simulink model "DQN_ABC_Test"  (R2023b)
settings: Solver=ode23tb  StartTime=0.0  StopTime=0.1  FixedStep=Ts  RelTol=1e-3
values from neighbouring files (symbols this model uses):
  Carm = 3.76    [DQn_ABC_Test_calc.m]
  L = Ld + Lm    [DQn_ABC_Test_calc.m]
  La = 1e-3    (= 0.001)    [DQn_ABC_Test_calc.m]
  Lb = 2*La    (= 0.002)    [DQn_ABC_Test_calc.m]
  Lc = 0.5*La    (= 0.0005)    [DQn_ABC_Test_calc.m]
  N = 1    [DQn_ABC_Test_calc.m]
  R = Rd + Rm    [DQn_ABC_Test_calc.m]
  Ra = 1.64    [DQn_ABC_Test_calc.m]
  Rb = 1.4*Ra    (= 2.296)    [DQn_ABC_Test_calc.m]
  Rc = 2.8*Ra    (= 4.592)    [DQn_ABC_Test_calc.m]
  Ta_dqn = oDP.Ta_dqn    [DQn_ABC_Test_calc.m]
  Ts = 50e-6    (= 5e-05)    [DQn_ABC_Test_calc.m]
  Ts_dqn = Ts    (= 5e-05)    [DQn_ABC_Test_calc.m]
  Ts_emt = Ts    (= 5e-05)    [DQn_ABC_Test_calc.m]
  Ws = 2*pi*f    (= 314.159265359)    [DQn_ABC_Test_calc.m]
undefined symbols (not defined in the file or in its folder): DiscIntNeverNeededParam, i, Xdcpnz, Xdcpnz_c, Xpnz, Ydcpnz, Ydcpnz_c, Ypnz
libraries: DQN_Lib x81, spsCurrentMeasurementLib x9, spsControlledVoltageSourceLib x9, spsSeriesRLCBranchLib x6, spsGroundLib x6, simulink x3, spsMutualInductanceLib x1, spspowerguiLib x1
(part 2 of 6)

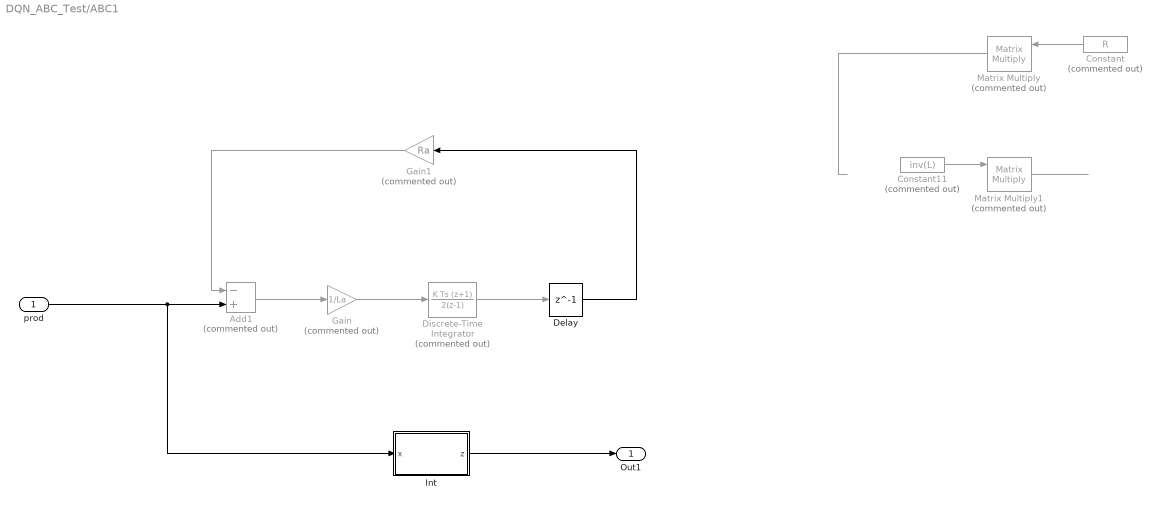
== system DQN_ABC_Test/ABC1 ==
  prod : Inport
  Add1 : Sum  Commented=on  Inputs=-+
  Constant : Constant  Commented=on  Value=R
  Constant11 : Constant  Commented=on  Value=inv(L)
  Delay : Delay  DelayLength=1
  Discrete-Time Integrator : DiscreteIntegrator  Commented=on  IntegratorMethod=Integration: Trapezoidal  SampleTime=Ts_emt  ICPrevOutput=DiscIntNeverNeededParam  ICPrevScaledInput=DiscIntNeverNeededParam
  Gain : Gain  Commented=on  Gain=1/La
  Gain1 : Gain  Commented=on  Gain=Ra
  Int : MATLAB Function  TreatAsAtomicUnit=on  mask{dt=Ts_emt}
      mask prompts: dt "Time step (s):"
  Matrix Multiply : Product  Commented=on  Multiplication=Matrix(*)
  Matrix Multiply1 : Product  Commented=on  Multiplication=Matrix(*)
  Out1 : Outport
  wires:
  prod/1 -> Int/1(x), Add1/2
  ? -> Matrix Multiply1/2
  Constant11/1 -> Matrix Multiply1/1
  Constant/1 -> Matrix Multiply/1
  Matrix Multiply1/1 -> ?
  Matrix Multiply/1 -> ?
  ? -> Matrix Multiply/2
  Add1/1 -> Gain/1
  Int/1(z) -> Out1/1
  Gain1/1 -> Add1/1
  Gain/1 -> Discrete-Time Integrator/1
  Discrete-Time Integrator/1 -> Delay/1
  Delay/1 -> Gain1/1

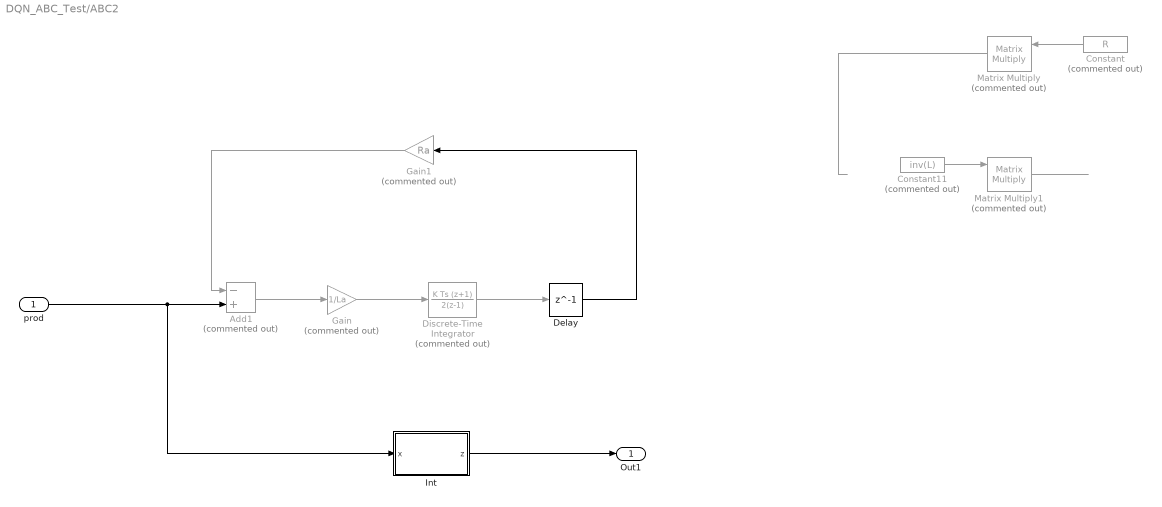
== system DQN_ABC_Test/ABC2 ==
  prod : Inport
  Add1 : Sum  Commented=on  Inputs=-+
  Constant : Constant  Commented=on  Value=R
  Constant11 : Constant  Commented=on  Value=inv(L)
  Delay : Delay  DelayLength=1
  Discrete-Time Integrator : DiscreteIntegrator  Commented=on  IntegratorMethod=Integration: Trapezoidal  SampleTime=Ts_emt  ICPrevOutput=DiscIntNeverNeededParam  ICPrevScaledInput=DiscIntNeverNeededParam
  Gain : Gain  Commented=on  Gain=1/La
  Gain1 : Gain  Commented=on  Gain=Ra
  Int : MATLAB Function  TreatAsAtomicUnit=on  mask{dt=Ts_emt}
      mask prompts: dt "Time step (s):"
  Matrix Multiply : Product  Commented=on  Multiplication=Matrix(*)
  Matrix Multiply1 : Product  Commented=on  Multiplication=Matrix(*)
  Out1 : Outport
  wires:
  prod/1 -> Int/1(x), Add1/2
  ? -> Matrix Multiply1/2
  Constant11/1 -> Matrix Multiply1/1
  Constant/1 -> Matrix Multiply/1
  Matrix Multiply1/1 -> ?
  Matrix Multiply/1 -> ?
  ? -> Matrix Multiply/2
  Add1/1 -> Gain/1
  Int/1(z) -> Out1/1
  Gain1/1 -> Add1/1
  Gain/1 -> Discrete-Time Integrator/1
  Discrete-Time Integrator/1 -> Delay/1
  Delay/1 -> Gain1/1

== system DQN_ABC_Test/DQN ==
  Y_DQN : Inport
  Add : Sum
  Delay1 : Delay  DelayLength=1  SampleTime=Ts_dqn
  Gain : Gain  Gain=1/La
  Gain1 : Gain  Gain=Ra
  Gain2 : Gain  Gain=-1
  sInt_DQN_fdbk : DQN_Lib/sInt_DQN_fdbk  HRM=N  Ws=Ws  Ts=Ts_dqn  HrmSeq=off  swFeed=off  R=Ra  iL=1/La
  Out1 : Outport
  wires:
  Delay1/1 -> Gain1/1, Out1/1
  Gain/1 -> sInt_DQN_fdbk/1
  Add/1 -> Gain/1
  sInt_DQN_fdbk/1 -> Delay1/1
  Gain1/1 -> Gain2/1
  Gain2/1 -> Add/1
  Y_DQN/1 -> Add/2

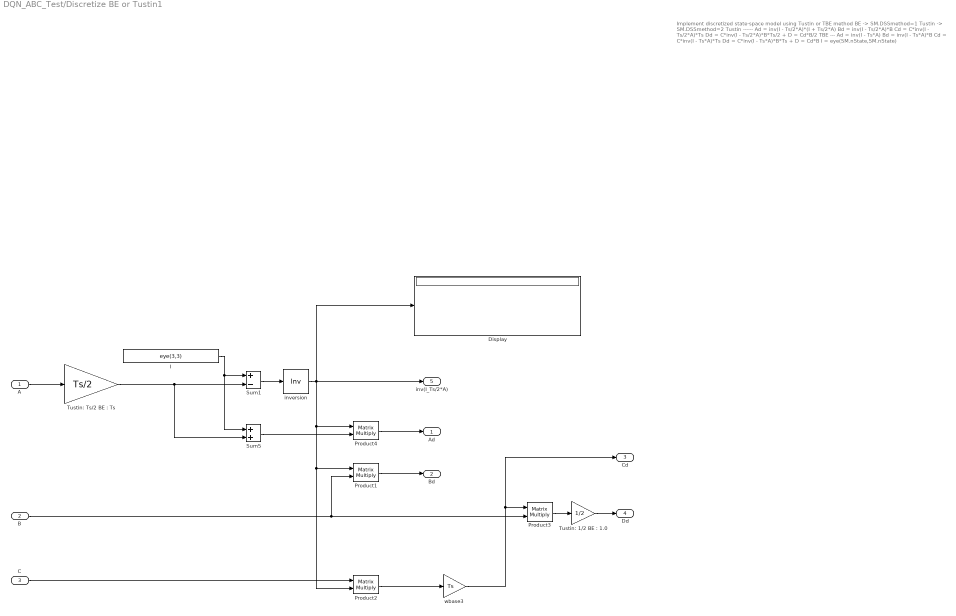
== system DQN_ABC_Test/Discretize BE or Tustin1 ==
  note: Implement discretized state-space model using Tustin or TBE method
      |
      | BE      -> SM.DSSmethod=1
      | Tustin  -> SM.DSSmethod=2
      |
      |
      | Tustin
      | ------
      | Ad = inv(I - Ts/2*A)*(I + Ts/2*A)
      | Bd = inv(I - Ts/2*A)*B
      | Cd = C*inv(I - Ts/2*A)*Ts
      | Dd = C*inv(I - Ts/2*A)*B*Ts/2  + D  =  Cd*B/2
      |
      | TBE
      | ---
      | Ad = inv(I - Ts*A)
      | Bd = inv(I - Ts*A)*B
      | Cd = C*inv(I - Ts*A)*Ts
      | Dd = C*inv(I - Ts*A)*B*Ts  + D  =  Cd*B
      |
      | I = eye(SM.nState,SM.nState)
  A : Inport
  B : Inport  Port=2
  C : Inport  Port=3
  Display : Display
  I : Constant  Value=eye(3,3)
  Product{1..4} (4 alike) : Product  Multiplication=Matrix(*)  SaturateOnIntegerOverflow=on  OutDataTypeStr=Inherit: Same as first input
  Sum1 : Sum  Inputs=+-  SaturateOnIntegerOverflow=on
  Sum5 : Sum  SaturateOnIntegerOverflow=on
  "Tustin: 1/2 BE : 1.0" : Gain  Gain=1/2  SaturateOnIntegerOverflow=on  OutDataTypeStr=Inherit: Same as input  ParamDataTypeStr=Inherit: Same as input
  "Tustin: Ts/2 BE : Ts" : Gain  Gain=Ts/2  SaturateOnIntegerOverflow=on  OutDataTypeStr=Inherit: Same as input  ParamDataTypeStr=Inherit: Same as input
  inversion : Product  Inputs=/  Multiplication=Matrix(*)  RndMeth=Zero
  wbase3 : Gain  Gain=Ts  SaturateOnIntegerOverflow=on  OutDataTypeStr=Inherit: Same as input  ParamDataTypeStr=Inherit: Same as input
  Ad : Outport  VectorParamsAs1DForOutWhenUnconnected=off
  Bd : Outport  Port=2  VectorParamsAs1DForOutWhenUnconnected=off
  Cd : Outport  Port=3  VectorParamsAs1DForOutWhenUnconnected=off
  Dd : Outport  Port=4  VectorParamsAs1DForOutWhenUnconnected=off
  inv(I_Ts/2*A) : Outport  Port=5  VectorParamsAs1DForOutWhenUnconnected=off
  wires:
  wbase3/1 -> Product3/1, Cd/1
  Product2/1 -> wbase3/1
  "Tustin: 1/2 BE : 1.0"/1 -> Dd/1
  Product3/1 -> "Tustin: 1/2 BE : 1.0"/1
  C/1 -> Product2/1
  B/1 -> Product3/2, Product1/2
  Product1/1 -> Bd/1
  Sum5/1 -> Product4/2
  inversion/1 -> Display/1, inv(I_Ts/2*A)/1, Product4/1, Product1/1, Product2/2
  Sum1/1 -> inversion/1
  I/1 -> Sum1/1, Sum5/1
  A/1 -> "Tustin: Ts/2 BE : Ts"/1
  Product4/1 -> Ad/1
  "Tustin: Ts/2 BE : Ts"/1 -> Sum5/2, Sum1/2

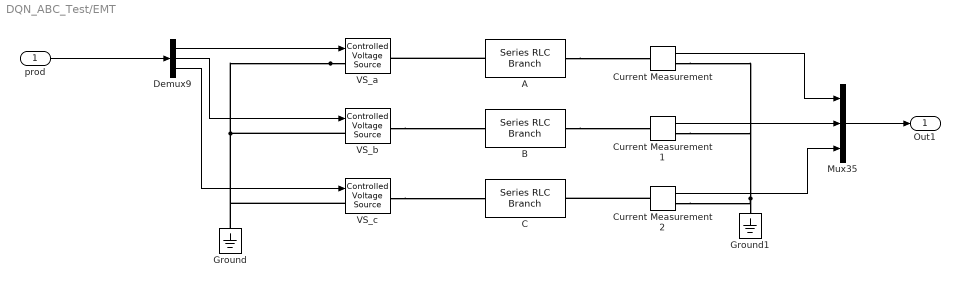
== system DQN_ABC_Test/EMT ==
  prod : Inport
  A : spsSeriesRLCBranchLib/Series RLC Branch  LConnTagsString=__new0  RConnTagsString=__new0  BranchType=RL  Resistance=Ra  Inductance=La  SetiL0=off  InitialCurrent=0  Capacitance=1e-6  Setx0=off  InitialVoltage=0  Measurements=None
  B : spsSeriesRLCBranchLib/Series RLC Branch  LConnTagsString=__new0  RConnTagsString=__new0  BranchType=RL  Resistance=Rb  Inductance=Lb  SetiL0=off  InitialCurrent=0  Capacitance=1e-6  Setx0=off  InitialVoltage=0  Measurements=None
  C : spsSeriesRLCBranchLib/Series RLC Branch  LConnTagsString=__new0  RConnTagsString=__new0  BranchType=RL  Resistance=Rc  Inductance=Lc  SetiL0=off  InitialCurrent=0  Capacitance=1e-6  Setx0=off  InitialVoltage=0  Measurements=None
  Current Measurement : spsCurrentMeasurementLib/Current Measurement  PhasorSimulation=off  OutputType=Complex  PSBequivalent=0
  Current Measurement1 : spsCurrentMeasurementLib/Current Measurement  PhasorSimulation=off  OutputType=Complex  PSBequivalent=0
  Current Measurement2 : spsCurrentMeasurementLib/Current Measurement  PhasorSimulation=off  OutputType=Complex  PSBequivalent=0
  Demux9 : Demux  Outputs=3
  Ground : spsGroundLib/Ground  LConnTagsString=a
  Ground1 : spsGroundLib/Ground  LConnTagsString=a
  Mux35 : Mux  Inputs=3
  VS_a : spsControlledVoltageSourceLib/Controlled Voltage Source  Initialize=on  Source_Type=AC  Amplitude=0  Phase=0  Frequency=0  Measurements=None
  VS_b : spsControlledVoltageSourceLib/Controlled Voltage Source  Initialize=on  Source_Type=AC  Amplitude=0  Phase=0  Frequency=0  Measurements=None
  VS_c : spsControlledVoltageSourceLib/Controlled Voltage Source  Initialize=on  Source_Type=AC  Amplitude=0  Phase=0  Frequency=0  Measurements=None
  Out1 : Outport
  wires:
  Current Measurement/1 -> Mux35/1
  Demux9/1 -> VS_a/1
  Demux9/2 -> VS_b/1
  Current Measurement2/1 -> Mux35/3
  Current Measurement1/1 -> Mux35/2
  Demux9/3 -> VS_c/1
  Mux35/1 -> Out1/1
  prod/1 -> Demux9/1
  connections:
  VS_a/LConn1 -- Ground/LConn1 -- VS_c/LConn1 -- VS_b/LConn1
  VS_b/RConn1 -- B/LConn1
  Ground1/LConn1 -- Current Measurement/RConn1 -- Current Measurement1/RConn1 -- Current Measurement2/RConn1
  A/RConn1 -- Current Measurement/LConn1
  VS_c/RConn1 -- C/LConn1
  Current Measurement2/LConn1 -- C/RConn1
  B/RConn1 -- Current Measurement1/LConn1
  A/LConn1 -- VS_a/RConn1

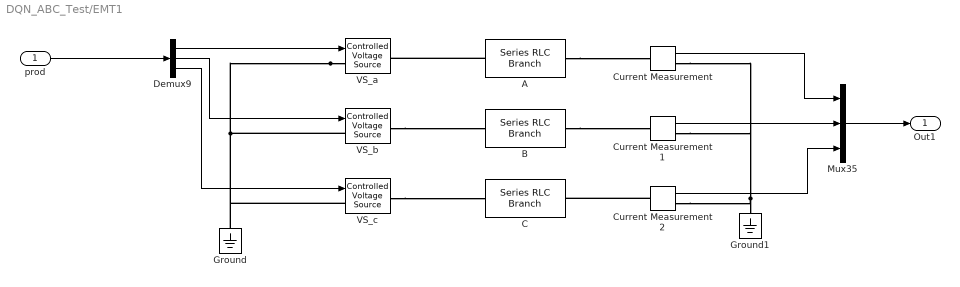
== system DQN_ABC_Test/EMT1 ==
  prod : Inport
  A : spsSeriesRLCBranchLib/Series RLC Branch  LConnTagsString=__new0  RConnTagsString=__new0  BranchType=RL  Resistance=Ra  Inductance=La  SetiL0=off  InitialCurrent=0  Capacitance=1e-6  Setx0=off  InitialVoltage=0  Measurements=None
  B : spsSeriesRLCBranchLib/Series RLC Branch  LConnTagsString=__new0  RConnTagsString=__new0  BranchType=RL  Resistance=Rb  Inductance=Lb  SetiL0=off  InitialCurrent=0  Capacitance=1e-6  Setx0=off  InitialVoltage=0  Measurements=None
  C : spsSeriesRLCBranchLib/Series RLC Branch  LConnTagsString=__new0  RConnTagsString=__new0  BranchType=RL  Resistance=Rc  Inductance=Lc  SetiL0=off  InitialCurrent=0  Capacitance=1e-6  Setx0=off  InitialVoltage=0  Measurements=None
  Current Measurement : spsCurrentMeasurementLib/Current Measurement  PhasorSimulation=off  OutputType=Complex  PSBequivalent=0
  Current Measurement1 : spsCurrentMeasurementLib/Current Measurement  PhasorSimulation=off  OutputType=Complex  PSBequivalent=0
  Current Measurement2 : spsCurrentMeasurementLib/Current Measurement  PhasorSimulation=off  OutputType=Complex  PSBequivalent=0
  Demux9 : Demux  Outputs=3
  Ground : spsGroundLib/Ground  LConnTagsString=a
  Ground1 : spsGroundLib/Ground  LConnTagsString=a
  Mux35 : Mux  Inputs=3
  VS_a : spsControlledVoltageSourceLib/Controlled Voltage Source  Initialize=on  Source_Type=AC  Amplitude=0  Phase=0  Frequency=0  Measurements=None
  VS_b : spsControlledVoltageSourceLib/Controlled Voltage Source  Initialize=on  Source_Type=AC  Amplitude=0  Phase=0  Frequency=0  Measurements=None
  VS_c : spsControlledVoltageSourceLib/Controlled Voltage Source  Initialize=on  Source_Type=AC  Amplitude=0  Phase=0  Frequency=0  Measurements=None
  Out1 : Outport
  wires:
  Current Measurement/1 -> Mux35/1
  Demux9/1 -> VS_a/1
  Demux9/2 -> VS_b/1
  Current Measurement2/1 -> Mux35/3
  Current Measurement1/1 -> Mux35/2
  Demux9/3 -> VS_c/1
  Mux35/1 -> Out1/1
  prod/1 -> Demux9/1
  connections:
  VS_a/LConn1 -- Ground/LConn1 -- VS_c/LConn1 -- VS_b/LConn1
  VS_b/RConn1 -- B/LConn1
  Ground1/LConn1 -- Current Measurement/RConn1 -- Current Measurement1/RConn1 -- Current Measurement2/RConn1
  A/RConn1 -- Current Measurement/LConn1
  VS_c/RConn1 -- C/LConn1
  Current Measurement2/LConn1 -- C/RConn1
  B/RConn1 -- Current Measurement1/LConn1
  A/LConn1 -- VS_a/RConn1

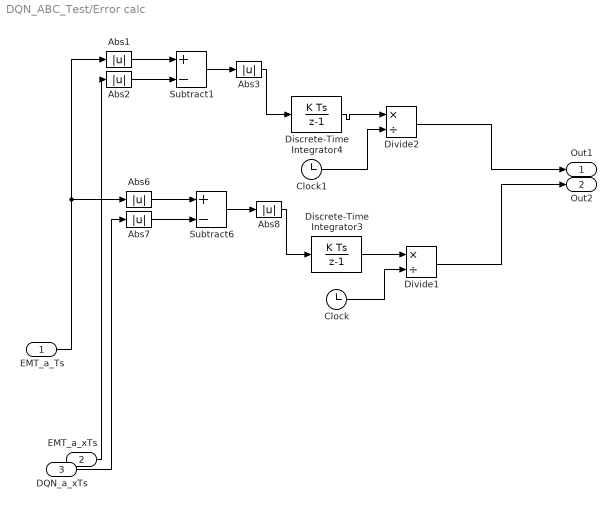
== system DQN_ABC_Test/Error calc ==
  EMT_a_Ts : Inport
  EMT_a_xTs : Inport  Port=2
  DQN_a_xTs : Inport  Port=3
  Abs{1..3,6..8} (6 alike) : Abs  ZeroCross=off  SaturateOnIntegerOverflow=off
  Clock : Clock
  Clock1 : Clock
  Discrete-Time Integrator3 : DiscreteIntegrator  SampleTime=Ts_dqn  ICPrevOutput=DiscIntNeverNeededParam  ICPrevScaledInput=DiscIntNeverNeededParam
  Discrete-Time Integrator4 : DiscreteIntegrator  SampleTime=Ts_dqn  ICPrevOutput=DiscIntNeverNeededParam  ICPrevScaledInput=DiscIntNeverNeededParam
  Divide1 : Product  Inputs=*/
  Divide2 : Product  Inputs=*/
  Subtract1 : Sum  Inputs=+-
  Subtract6 : Sum  Inputs=+-
  Out1 : Outport
  Out2 : Outport  Port=2
  wires:
  Abs2/1 -> Subtract1/2
  Clock/1 -> Divide1/2
  Clock1/1 -> Divide2/2
  Abs6/1 -> Subtract6/1
  Discrete-Time Integrator4/1 -> Divide2/1
  Discrete-Time Integrator3/1 -> Divide1/1
  Abs3/1 -> Discrete-Time Integrator4/1
  EMT_a_Ts/1 -> Abs1/1, Abs6/1
  Subtract1/1 -> Abs3/1
  Abs1/1 -> Subtract1/1
  DQN_a_xTs/1 -> Abs7/1
  EMT_a_xTs/1 -> Abs2/1
  Subtract6/1 -> Abs8/1
  Divide2/1 -> Out1/1
  Abs7/1 -> Subtract6/2
  Abs8/1 -> Discrete-Time Integrator3/1
  Divide1/1 -> Out2/1

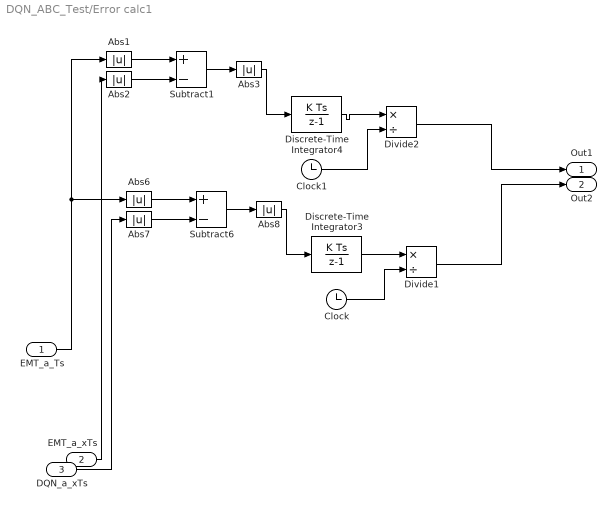
== system DQN_ABC_Test/Error calc1 ==
  EMT_a_Ts : Inport
  EMT_a_xTs : Inport  Port=2
  DQN_a_xTs : Inport  Port=3
  Abs{1..3,6..8} (6 alike) : Abs  ZeroCross=off  SaturateOnIntegerOverflow=off
  Clock : Clock
  Clock1 : Clock
  Discrete-Time Integrator3 : DiscreteIntegrator  SampleTime=Ts_dqn  ICPrevOutput=DiscIntNeverNeededParam  ICPrevScaledInput=DiscIntNeverNeededParam
  Discrete-Time Integrator4 : DiscreteIntegrator  SampleTime=Ts_dqn  ICPrevOutput=DiscIntNeverNeededParam  ICPrevScaledInput=DiscIntNeverNeededParam
  Divide1 : Product  Inputs=*/
  Divide2 : Product  Inputs=*/
  Subtract1 : Sum  Inputs=+-
  Subtract6 : Sum  Inputs=+-
  Out1 : Outport
  Out2 : Outport  Port=2
  wires:
  Abs2/1 -> Subtract1/2
  Clock/1 -> Divide1/2
  Clock1/1 -> Divide2/2
  Abs6/1 -> Subtract6/1
  Discrete-Time Integrator4/1 -> Divide2/1
  Discrete-Time Integrator3/1 -> Divide1/1
  Abs3/1 -> Discrete-Time Integrator4/1
  EMT_a_Ts/1 -> Abs1/1, Abs6/1
  Subtract1/1 -> Abs3/1
  Abs1/1 -> Subtract1/1
  DQN_a_xTs/1 -> Abs7/1
  EMT_a_xTs/1 -> Abs2/1
  Subtract6/1 -> Abs8/1
  Divide2/1 -> Out1/1
  Abs7/1 -> Subtract6/2
  Abs8/1 -> Discrete-Time Integrator3/1
  Divide1/1 -> Out2/1

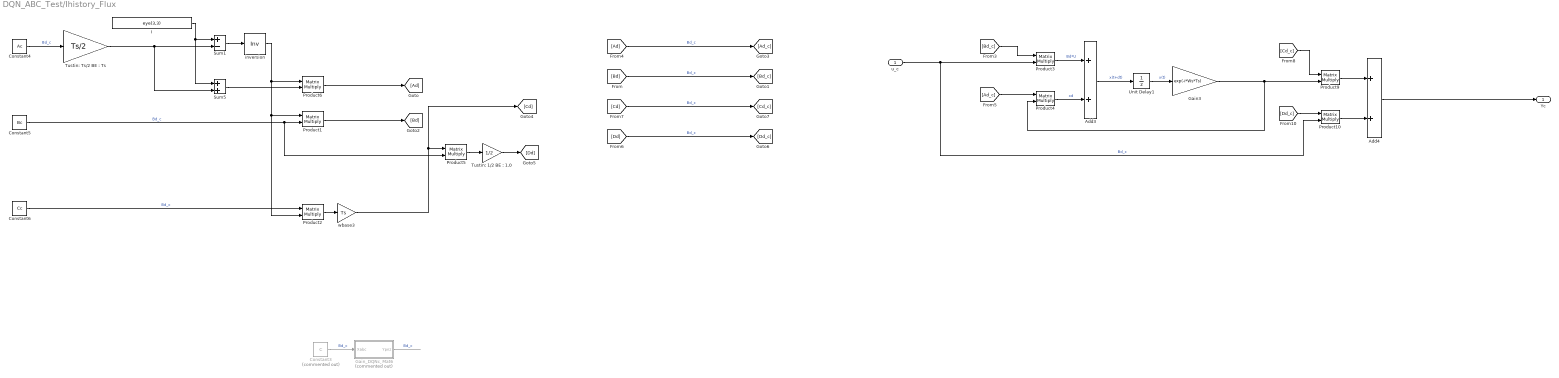
== system DQN_ABC_Test/Ihistory_Flux ==
  u_c : Inport
  Add3 : Sum
  Add4 : Sum
  Constant3 : Constant  Commented=on  Value=C
  Constant4 : Constant  Value=Ac
  Constant5 : Constant  Value=Bc
  Constant6 : Constant  Value=Cc
  Gain3 : Gain  Gain=exp(-i*Ws*Ts)
  Gain_DQNc_Mat6 : MATLAB Function  Commented=on  TreatAsAtomicUnit=on  SystemSampleTime=Ts  mask{Rabc=eye(3)/L, HRM=N, chkInv=off}
      mask prompts: Rabc "Line matrix [3x3]:"; HRM "Harmonic order:"; chkInv "Invert"
  I : Constant  Value=eye(3,3)
  Product{1..6,9..10} (8 alike) : Product  Multiplication=Matrix(*)  SaturateOnIntegerOverflow=on  OutDataTypeStr=Inherit: Same as first input
  Sum1 : Sum  Inputs=+-  SaturateOnIntegerOverflow=on
  Sum5 : Sum  SaturateOnIntegerOverflow=on
  "Tustin: 1/2 BE : 1.0" : Gain  Gain=1/2  SaturateOnIntegerOverflow=on  OutDataTypeStr=Inherit: Same as input  ParamDataTypeStr=Inherit: Same as input
  "Tustin: Ts/2 BE : Ts" : Gain  Gain=Ts/2  SaturateOnIntegerOverflow=on  OutDataTypeStr=Inherit: Same as input  ParamDataTypeStr=Inherit: Same as input
  Unit Delay1 : UnitDelay  SampleTime=Ts  HasFrameUpgradeWarning=on
  inversion : Product  Inputs=/  Multiplication=Matrix(*)  RndMeth=Zero
  wbase3 : Gain  Gain=Ts  SaturateOnIntegerOverflow=on  OutDataTypeStr=Inherit: Same as input  ParamDataTypeStr=Inherit: Same as input
  Yc : Outport  VectorParamsAs1DForOutWhenUnconnected=off
  wires:
  [Bd] -> [Bd_c]  "Bd_c"
  [Bd_c] -> Product3/1
  [Ad] -> [Ad_c]  "Bd_c"
  [Ad_c] -> Product4/1
  Product3/1 -> Add3/1  "Bd*U"
  [Cd] -> [Cd_c]  "Bd_c"
  [Dd] -> [Dd_c]  "Bd_c"
  u_c/1 -> Product10/2, Product3/2  "Bd_c"
  Unit Delay1/1 -> Gain3/1  "x(t)"
  Add3/1 -> Unit Delay1/1  "x(t+dt)"
  Product4/1 -> Add3/2  "xd"
  [Cd_c] -> Product9/1
  [Dd_c] -> Product10/1
  Product9/1 -> Add4/1
  Product10/1 -> Add4/2
  inversion/1 -> Product6/1, Product1/1, Product2/2
  Sum1/1 -> inversion/1
  "Tustin: Ts/2 BE : Ts"/1 -> Sum5/2, Sum1/2
  Product5/1 -> "Tustin: 1/2 BE : 1.0"/1
  Sum5/1 -> Product6/2
  I/1 -> Sum1/1, Sum5/1
  "Tustin: 1/2 BE : 1.0"/1 -> [Dd]
  Product2/1 -> wbase3/1
  Product6/1 -> [Ad]
  Product1/1 -> [Bd]
  wbase3/1 -> [Cd], Product5/1
  Constant3/1 -> Gain_DQNc_Mat6/1(Xabc)  "Bd_c"
  Constant4/1 -> "Tustin: Ts/2 BE : Ts"/1  "Bd_c"
  Constant5/1 -> Product5/2, Product1/2  "Bd_c"
  Gain_DQNc_Mat6/1(Ypnz) -> ?  "Bd_c"
  Constant6/1 -> Product2/1  "Bd_c"
  Add4/1 -> Yc/1
  Gain3/1 -> Product9/2, Product4/2

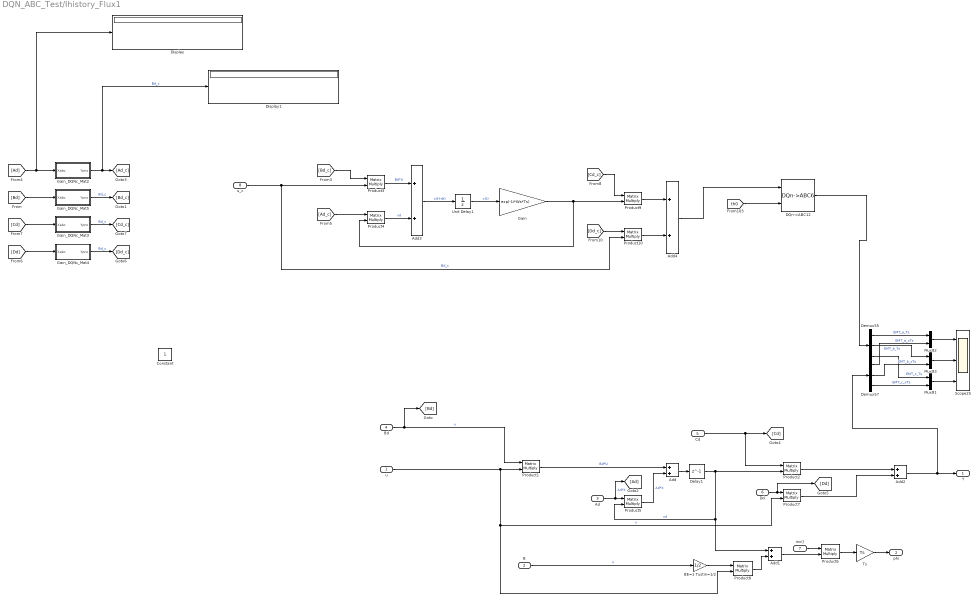
== system DQN_ABC_Test/Ihistory_Flux1 ==
  u : Inport
  B : Inport  Port=2
  Ad : Inport  Port=3
  Bd : Inport  Port=4
  Cd : Inport  Port=5
  Dd : Inport  Port=6
  inv() : Inport  Port=7
  u_c : Inport  Port=8
  Add{,1..4} (5 alike) : Sum
  BE=1 Tustin=1/2 : Gain  Gain=1/2
  Constant : Constant
  DQn->ABC12 : DQN_Lib/DQn->ABC6  N=N
  Delay1 : Delay  DelayLength=1  SampleTime=Ts
  Demux55 : Demux  Outputs=3
  Demux57 : Demux  Outputs=3
  Display : Display
  Display1 : Display
  Gain : Gain  Gain=exp(-1i*Ws*Ts)
  Gain_DQNc_Mat2 : MATLAB Function  TreatAsAtomicUnit=on  SystemSampleTime=Ts  mask{Rabc=eye(3)/L, HRM=N, chkInv=off}
      mask prompts: Rabc "Line matrix [3x3]:"; HRM "Harmonic order:"; chkInv "Invert"
  Gain_DQNc_Mat3 : MATLAB Function  TreatAsAtomicUnit=on  SystemSampleTime=Ts  mask{Rabc=eye(3)/L, HRM=N, chkInv=off}
      mask prompts: Rabc "Line matrix [3x3]:"; HRM "Harmonic order:"; chkInv "Invert"
  Gain_DQNc_Mat4 : MATLAB Function  TreatAsAtomicUnit=on  SystemSampleTime=Ts  mask{Rabc=eye(3)/L, HRM=N, chkInv=off}
      mask prompts: Rabc "Line matrix [3x3]:"; HRM "Harmonic order:"; chkInv "Invert"
  Gain_DQNc_Mat5 : MATLAB Function  TreatAsAtomicUnit=on  SystemSampleTime=Ts  mask{Rabc=eye(3)/L, HRM=N, chkInv=off}
      mask prompts: Rabc "Line matrix [3x3]:"; HRM "Harmonic order:"; chkInv "Invert"
  Mux81 : Mux  Inputs=2
  Mux82 : Mux  Inputs=2
  Mux83 : Mux  Inputs=2
  Product{1..10} (10 alike) : Product  Multiplication=Matrix(*)  SaturateOnIntegerOverflow=on  OutDataTypeStr=Inherit: Same as first input
  Scope25 : Scope  NumInputPorts=3
  Ts : Gain  Gain=Ts  SaturateOnIntegerOverflow=on  OutDataTypeStr=Inherit: Same as input  ParamDataTypeStr=Inherit: Same as input
  Unit Delay1 : UnitDelay  SampleTime=Ts  HasFrameUpgradeWarning=on
  Y : Outport  VectorParamsAs1DForOutWhenUnconnected=off
  phi : Outport  Port=2  VectorParamsAs1DForOutWhenUnconnected=off
  wires:
  Ts/1 -> phi/1
  Add2/1 -> Demux57/1, Y/1
  B/1 -> BE=1 Tustin=1/2/1  "u"
  Bd/1 -> [Bd], Product1/1  "u"
  u/1 -> Product7/2, Product8/2, Product1/2  "u"
  Dd/1 -> [Dd], Product7/1
  Product7/1 -> Add2/2
  Product2/1 -> Add2/1
  Product1/1 -> Add/1  "Bd*U"
  Add/1 -> Delay1/1
  Delay1/1 -> Product5/2, Add1/1, Product2/2  "xd"
  Ad/1 -> [Ad], Product5/1  "Ad*X"
  Product6/1 -> Ts/1
  Product8/1 -> Add1/2
  Add1/1 -> Product6/2
  Cd/1 -> [Cd], Product2/1
  inv()/1 -> Product6/1
  BE=1 Tustin=1/2/1 -> Product8/1
  [th0] -> DQn->ABC12/2
  Demux57/1 -> Mux82/2  "EMT_a_xTs"
  Mux83/1 -> Scope25/2
  Demux57/2 -> Mux83/2  "EMT_b_xTs"
  Demux57/3 -> Mux81/2  "EMT_c_xTs"
  Mux82/1 -> Scope25/1
  Mux81/1 -> Scope25/3
  Demux55/1 -> Mux82/1  "EMT_a_Ts"
  Demux55/2 -> Mux83/1  "EMT_b_Ts"
  Demux55/3 -> Mux81/1  "EMT_c_Ts"
  DQn->ABC12/1 -> Demux55/1
  [Bd] -> Gain_DQNc_Mat5/1(Xabc)
  Gain_DQNc_Mat5/1(Ypnz) -> [Bd_c]  "Bd_c"
  [Bd_c] -> Product3/1
  Gain_DQNc_Mat2/1(Ypnz) -> Display1/1, [Ad_c]  "Bd_c"
  [Ad] -> Display/1, Gain_DQNc_Mat2/1(Xabc)
  [Ad_c] -> Product4/1
  Product3/1 -> Add3/1  "Bd*U"
  Gain_DQNc_Mat3/1(Ypnz) -> [Cd_c]  "Bd_c"
  Gain_DQNc_Mat4/1(Ypnz) -> [Dd_c]  "Bd_c"
  [Cd] -> Gain_DQNc_Mat3/1(Xabc)
  [Dd] -> Gain_DQNc_Mat4/1(Xabc)
  Product5/1 -> Add/2  "Ad*X"
  u_c/1 -> Product10/2, Product3/2  "Bd_c"
  Unit Delay1/1 -> Gain/1  "x(t)"
  Add3/1 -> Unit Delay1/1  "x(t+dt)"
  Product4/1 -> Add3/2  "xd"
  Gain/1 -> Product9/2, Product4/2
  [Cd_c] -> Product9/1
  [Dd_c] -> Product10/1
  Product9/1 -> Add4/1
  Product10/1 -> Add4/2
  Add4/1 -> DQn->ABC12/1

== system DQN_ABC_Test/Int_DQN_fdbk2 ==
  X_DQN : Inport
  Demux : Demux  Outputs=6
  Int_d_2N_2 : MATLAB Function  TreatAsAtomicUnit=on  mask{N=HrmOrd, dt=TimeStep, w=FreqRad, SW=swFeed, R=R, iL=iL}
      mask prompts: N "Order number:"; dt "Time step (s):"; w "Angular frequency (1/rad):"; SW "Enable feedback"; R "Feedback parameter (Kr):"; iL "Integrator parameter (Kl):"
  Mux51 : Mux  Inputs=[(1)*HrmOrd+1,(1)*HrmOrd+1,(1)*HrmOrd+1,(1)*HrmOrd+1,(1)*HrmOrd+1,(1)*HrmOrd+1]
  Z_DQN : Outport
  wires:
  X_DQN/1 -> Demux/1
  Mux51/1 -> Z_DQN/1
  Demux/3 -> Int_d_2N_2/3(Xdz)
  Demux/2 -> Int_d_2N_2/2(Xdn)
  Demux/4 -> Int_d_2N_2/4(Xqp)
  Demux/1 -> Int_d_2N_2/1(Xdp)
  Demux/5 -> Int_d_2N_2/5(Xqn)
  Demux/6 -> Int_d_2N_2/6(Xqz)
  Int_d_2N_2/3(Zdz) -> Mux51/3
  Int_d_2N_2/2(Zdn) -> Mux51/2
  Int_d_2N_2/4(Zqp) -> Mux51/4
  Int_d_2N_2/1(Zdp) -> Mux51/1
  Int_d_2N_2/5(Zqn) -> Mux51/5
  Int_d_2N_2/6(Zqz) -> Mux51/6

== system DQN_ABC_Test/Mux_DQNc_Mat ==
  In1 : Inport
  In2 : Inport  Port=2
  Mux : Concatenate  Mode=Multidimensional array
  Out1 : Outport
  wires:
  In1/1 -> Mux/1
  In2/1 -> Mux/2
  Mux/1 -> Out1/1

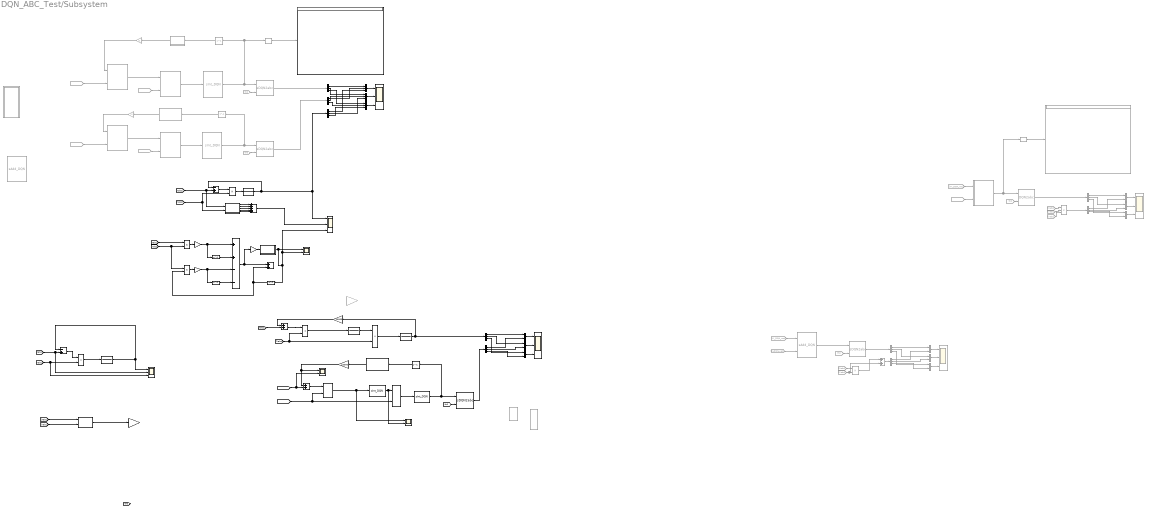
== system DQN_ABC_Test/Subsystem ==
  Add : Sum  Commented=on
  Add10 : Sum  Inputs=++--
  Add11 : Sum
  Add5 : Sum  Inputs=-+
  Add7 : Sum  Inputs=+++++
  DQN2abc5 : DQN_Lib/DQN2abc  Commented=on  HrmOrd=4*N
  Delay : Delay  Commented=on  DelayLength=1  SampleTime=Ts
  Delay1 : Delay  Commented=on  DelayLength=1  SampleTime=Ts
  Delay{2..5} (4 alike) : Delay  DelayLength=1  SampleTime=Ts
  Demux{8..9,16..17} (4 alike) : Demux  Commented=on  Outputs=3
  Demux{18,21,28..30} (5 alike) : Demux  Outputs=3
  Discrete-Time Integrator{3..6} (4 alike) : DiscreteIntegrator  IntegratorMethod=Integration: Trapezoidal  SampleTime=Ts  ICPrevOutput=DiscIntNeverNeededParam  ICPrevScaledInput=DiscIntNeverNeededParam
  Display : Display
  Display1 : Display  Commented=on
  From : From  Commented=on  GotoTag=XY_DQN_vec
  From17 : From  Commented=on  GotoTag=Xabc
  From{18,34,45,52} (4 alike) : From  Commented=on  GotoTag=Y_DQN_vec
  From21 : From  Commented=on  GotoTag=th0
  From22 : From  Commented=on  GotoTag=Yabc
  From24 : From  Commented=on  GotoTag=XY_DQN_vec
  From30 : From  Commented=on  GotoTag=Yabc
  From33 : From  Commented=on  GotoTag=th0
  From35 : From  Commented=on  GotoTag=Xabc
  From36 : From  Commented=on  GotoTag=Yabc
  From44 : From  Commented=on  GotoTag=X_DQN_vec
  From48 : From  Commented=on  GotoTag=th0  TagVisibility=global
  From50 : From  Commented=on  GotoTag=X_DQN_vec
  From53 : From  Commented=on  GotoTag=th0  TagVisibility=global
  Gain1 : Gain  Gain=Ts/2
  Gain2 : Gain  Commented=on  Gain=-1
  Gain3 : Gain  Commented=on  Gain=-1
  Gain34 : Gain  Gain=10000
  Gain4 : Gain  Gain=Ts/2
  Gain5 : Gain  Gain=1/Ts
  Gain6 : Gain  Commented=on  Gain=1/(Carm)
  Gain7 : Gain  Gain=10000
  Gain9 : Gain  Gain=1/(Carm)
  Int : MATLAB Function  TreatAsAtomicUnit=on  mask{dt=Ts}
      mask prompts: dt "Time step (s):"
  MATLAB Function : MATLAB Function  Commented=on  TreatAsAtomicUnit=on  mask{hIn=2*N, hOut=N}
      mask prompts: hIn "HRM input:"; hOut "HRM output:"
  MATLAB Function1 : MATLAB Function  TreatAsAtomicUnit=on
  MATLAB Function2 : MATLAB Function  TreatAsAtomicUnit=on
  Mult_DQN2 : Subsystem  Commented=on  mask{HrmOrd=2*N, HrmDbl=on, chkHrmLst=off, HrmLstX=[0 7 8], HrmLstY=[0 7 8]}
      mask prompts: HrmOrd "Harmonic order:"; HrmDbl "Double harmonic"; chkHrmLst "Only specific harmonics"; HrmLstX "Harmonic list X:"; HrmLstY "Harmonic list Y:"
      mask Callback chkHrmLst:
      | EMT = get_param(gcb,'chkHrmLst');
      | 
      | if(strcmp(EMT,'on'))
      |    set_param(gcb,'MaskVisibilities',{'on','on','on','on','on'});
      | else
      |    set_param(gcb,'MaskVisibilities',{'on','on','on','off','off'});
      | end
      mask Display:
      | %plot([0 1])
      | port_label('input',1,'{X}');
      | port_label('input',2,'{Y}');
      | port_label('output',1,'{Z}');
      | 
      | 
      | 
      | harm = str2num(get_param(gcb, 'HrmOrd'));
      | HrmDbl = get_param(gcb, 'HrmDbl');
      | if(HrmDbl=="on")
      |     disp(['{\color{black}\bf\fontsize{12}Hi:',num2str(harm),'}',newline,'{\color{red}\bf\fontsize{12}\{X\}}',newline,'{\color{black}\bf\fontsize{12}Ho:',num2str(2*harm),'}'], 'texmode','on');
      | else
      |     disp(['{\color{black}\bf\fontsize{12}Hi:',num2str(harm),'}',newline,'{\color{red}\bf\fontsize{12}\{X\}}',newline,'{\color{black}\bf\fontsize{12}Ho:',num2str(harm),'}'], 'texmode','on');
      | end
      | 
      | 
      | %text(.95,.05,[newline,'{\bf\fontsize{12}H=',harm,'}'], 'horizontalAlignment', 'right', 'verticalAlignment','bottom','texmode','on')
  Mult_DQN3 : DQN_Lib/Mult_DQN  HrmOrd=N  HrmDbl=on  chkHrmLst=off  HrmLstX=[0 7 8]  HrmLstY=[0 7 8]
  Mult_DQN4 : DQN_Lib/Mult_DQN  HrmOrd=2*N  HrmDbl=on  chkHrmLst=off  HrmLstX=[0 7 8]  HrmLstY=[0 7 8]
  Mux{13..14,18,23..25} (6 alike) : Mux  Commented=on  Inputs=2
  Mux28 : Mux  Inputs=3
  Mux29 : Mux  Inputs=3
  Mux31 : Mux  Inputs=3
  Mux37 : Mux  Inputs=2
  Mux38 : Mux  Inputs=2
  Mux39 : Mux  Inputs=2
  Product10 : Product  Commented=on  Inputs=3
  Product{17..22} (6 alike) : Product
  Product8 : Product  Commented=on
  Reshape : Reshape  Commented=on  OutputDimensionality=Customize  OutputDimensions=[2*N+1,6]
  Reshape5 : Reshape  Commented=on  OutputDimensionality=Customize  OutputDimensions=[4*N+1,6]
  Scope10 : Scope  NumInputPorts=2
  Scope11 : Scope  NumInputPorts=3
  Scope12 : Scope  NumInputPorts=2
  Scope13 : Scope  NumInputPorts=3
  Scope14 : Scope  NumInputPorts=2
  Subsystem1 : Subsystem  Commented=on  mask{Hi=N, Ho=N}
      mask prompts: Hi "Input harmonic order:"; Ho "Output harmonic order:"
  Subsystem2 : Subsystem  Commented=on  mask{Hi=2*N, Ho=N}
      mask prompts: Hi "Input harmonic order:"; Ho "Output harmonic order:"
  Subsystem3 : Subsystem  mask{Hi=4*N, Ho=N}
      mask prompts: Hi "Input harmonic order:"; Ho "Output harmonic order:"
  Subtract : Sum  Inputs=-+
  Subtract1 : Sum
  Subtract2 : Sum
  XY2 : Scope  Commented=on  NumInputPorts=3
  XY4 : Scope  NumInputPorts=3
  XY6 : Scope  Commented=on  NumInputPorts=3
  XY7 : Scope  NumInputPorts=3
  sAdd_DQN : DQN_Lib/sAdd_DQN  Commented=on  HRM=2*N
  sAdd_DQN1 : DQN_Lib/sAdd_DQN  Commented=on  HRM=N
  sAdd_DQN2 : Subsystem  Commented=on  mask{HRM=N}
      mask prompts: HRM "Harmonic order:"
      mask Display:
      | %plot([0 1])
      | port_label('input',1,'{X}');
      | port_label('input',2,'{Y}');
      | port_label('output',1,'{Z}');
      | 
      | 
      | 
      | %harm = (get_param(gcb, 'HRM'));
      | %disp(['{\color{black}\bf\fontsize{12}Hi:',num2str(harm),'}',newline,'{\color{red}\bf\fontsize{12}\{+\}}',newline,'{\color{black}\bf\fontsize{12}Ho:',num2str(harm),newline,'{\color{blue}\bf\fontsize{12}MEX}','}'], 'texmode','on');
      | harm = get_param(gcb, 'HRM');
      | disp(['{\color{black}\bf\fontsize{12}Hi:',(harm),'}',newline,'{\color{red}\bf\fontsize{12}\{+\}}',newline,'{\color{black}\bf\fontsize{12}Ho:',(harm),newline,'{\color{blue}\bf\fontsize{12}MEX}','}'], 'texmode','on');
  sAdd_DQN3 : Subsystem  Commented=on  mask{HRM=N}
      mask prompts: HRM "Harmonic order:"
      mask Display:
      | %plot([0 1])
      | port_label('input',1,'{X}');
      | port_label('input',2,'{Y}');
      | port_label('output',1,'{Z}');
      | 
      | 
      | 
      | %harm = (get_param(gcb, 'HRM'));
      | %disp(['{\color{black}\bf\fontsize{12}Hi:',num2str(harm),'}',newline,'{\color{red}\bf\fontsize{12}\{+\}}',newline,'{\color{black}\bf\fontsize{12}Ho:',num2str(harm),newline,'{\color{blue}\bf\fontsize{12}MEX}','}'], 'texmode','on');
      | harm = get_param(gcb, 'HRM');
      | disp(['{\color{black}\bf\fontsize{12}Hi:',(harm),'}',newline,'{\color{red}\bf\fontsize{12}\{+\}}',newline,'{\color{black}\bf\fontsize{12}Ho:',(harm),newline,'{\color{blue}\bf\fontsize{12}MEX}','}'], 'texmode','on');
  sDQN2abc10 : DQN_Lib/sDQN2abc  HRM=4*N
  sDQN2abc3 : DQN_Lib/sDQN2abc  Commented=on  HRM=2*N
  sDQN2abc8 : DQN_Lib/sDQN2abc  Commented=on  HRM=2*N
  sDQN2abc9 : DQN_Lib/sDQN2abc  Commented=on  HRM=N
  sInt_DQN1 : DQN_Lib/sInt_DQN  Commented=on  HRM=2*N  Ws=Ws  Ts=Ts  HrmSeq=off
  sInt_DQN2 : DQN_Lib/sInt_DQN  Commented=on  HRM=N  Ws=Ws  Ts=Ts  HrmSeq=off
  sInt_DQN3 : DQN_Lib/sInt_DQN  HRM=4*N  Ws=Ws  Ts=Ts  HrmSeq=off
  sInt_DQN4 : DQN_Lib/sInt_DQN  HRM=2*N  Ws=Ws  Ts=Ts  HrmSeq=off
  sMult_DQN2 : Subsystem  Commented=on  mask{HRM=N, HrmDbl=on, HrmSeq=off}
      mask prompts: HRM "Harmonic order:"; HrmDbl "Double harmonic"; HrmSeq "Pos. odd / neg. even harmonics (1p, 2n, 3p...)"
      mask init:
      | if(HrmDbl == 0 && HrmSeq == 0)
      |     HrmOpt = 0;
      | elseif(HrmDbl == 1 && HrmSeq == 0)
      |     HrmOpt = 1;
      | elseif(HrmDbl == 0 && HrmSeq == 1)
      |     HrmOpt = 2;
      | elseif(HrmDbl == 1 && HrmSeq == 1)
      |     HrmOpt = 3;
      | end
      mask Display:
      | %plot([0 1])
      | %port_label('input',1,'{X}');
      | %port_label('input',2,'{Y}');
      | %port_label('output',1,'{Z}');
      | 
      | port_label('input',1,'');
      | port_label('input',2,'');
      | port_label('output',1,'');
      | 
      | 
      | harm = str2num(get_param(gcb, 'HRM'));
      | HrmDbl = get_param(gcb, 'HrmDbl');
      | if(HrmDbl=="on")
      |     disp(['{\color{black}\bf\fontsize{12}Hi:',num2str(harm),'}',newline,'{\color{red}\bf\fontsize{12}\{X\}}',newline,'{\color{black}\bf\fontsize{12}Ho:',num2str(2*harm),newline,'{\color{blue}\bf\fontsize{12}MEX}','}'], 'texmode','on');
      | else
      |     disp(['{\color{black}\bf\fontsize{12}Hi:',num2str(harm),'}',newline,'{\color{red}\bf\fontsize{12}\{X\}}',newline,'{\color{black}\bf\fontsize{12}Ho:',num2str(harm),newline,'{\color{orange}\bf\fontsize{12}MEX}','}'], 'texmode','on');
      | end
      | 
      | %disp([newline,newline,newline,newline,newline,'{\color{black}\bf\fontsize{12}MEX}'],  'texmode','on');
      | 
      | 
      | 
      | %text(.95,.05,[newline,'{\bf\fontsize{12}H=',harm,'}'], 'horizontalAlignment', 'right', 'verticalAlignment','bottom','texmode','on')
  sMult_DQN3 : Subsystem  Commented=on  mask{HRM=N, HrmDbl=off, HrmSeq=off}
      mask prompts: HRM "Harmonic order:"; HrmDbl "Double harmonic"; HrmSeq "Pos. odd / neg. even harmonics (1p, 2n, 3p...)"
      mask init: same as DQN_ABC_Test/Subsystem/sMult_DQN2
      mask Display:
      | %plot([0 1])
      | %port_label('input',1,'{X}');
      | %port_label('input',2,'{Y}');
      | %port_label('output',1,'{Z}');
      | 
      | port_label('input',1,'');
      | port_label('input',2,'');
      | port_label('output',1,'');
      | 
      | 
      | harm = str2num(get_param(gcb, 'HRM'));
      | HrmDbl = get_param(gcb, 'HrmDbl');
      | if(HrmDbl=="on")
      |     disp(['{\color{black}\bf\fontsize{12}Hi:',num2str(harm),'}',newline,'{\color{red}\bf\fontsize{12}\{X\}}',newline,'{\color{black}\bf\fontsize{12}Ho:',num2str(2*harm),newline,'{\color{blue}\bf\fontsize{12}MEX}','}'], 'texmode','on');
      | else
      |     disp(['{\color{black}\bf\fontsize{12}Hi:',num2str(harm),'}',newline,'{\color{red}\bf\fontsize{12}\{X\}}',newline,'{\color{black}\bf\fontsize{12}Ho:',num2str(harm),newline,'{\color{orange}\bf\fontsize{12}MEX}','}'], 'texmode','on');
      | end
      | 
      | %disp([newline,newline,newline,newline,newline,'{\color{black}\bf\fontsize{12}MEX}'],  'texmode','on');
      | 
      | 
      | 
      | %text(.95,.05,[newline,'{\bf\fontsize{12}H=',harm,'}'], 'horizontalAlignment', 'right', 'verticalAlignment','bottom','texmode','on')
  sMult_DQN4 : DQN_Lib/sMult_DQN  Commented=on  HRM=2*N  HrmDbl=on  HrmSeq=off
  sMult_DQN5 : DQN_Lib/sMult_DQN  Commented=on  HRM=N  HrmDbl=on  HrmSeq=off
  wires:
  Subtract2/1 -> Mult_DQN3/1
  [X_DQN_vec] -> Subtract2/2, Scope12/2  "prod"
  Demux29/2 -> Mux38/2  "Product_b_ref"
  sDQN2abc10/1 -> Demux29/1  "prod"
  Demux28/3 -> Mux31/3  "Product_c_ref"
  [Yabc] -> Product18/2, Product19/2
  From45/1 -> sMult_DQN2/2(In2)
  [Xabc] -> Scope13/2, Subtract/2  "prod"
  Subsystem1/1("{Y_DQN}") -> Gain3/1
  Gain34/1 -> Subtract2/1, Scope12/1  "dVp_M"
  sInt_DQN3/1 -> Delay5/1, sDQN2abc10/1  "Vp_M"
  Demux28/2 -> Mux29/3  "Product_b_ref"
  Mux39/1 -> XY7/3
  sDQN2abc9/1 -> Demux18/1
  [Yabc] -> MATLAB Function2/2(y)
  Mult_DQN3/1 -> Scope14/1, sInt_DQN4/1  "dVp_M"
  Mult_DQN4/1 -> sInt_DQN3/1
  sAdd_DQN3/1(Out1) -> sMult_DQN3/1(In1)
  Product17/1 -> Discrete-Time Integrator3/1  "prod"
  Demux30/3 -> Mux39/1  "Product_c_proposed"
  Subtract1/1 -> Product18/1
  Mux38/1 -> XY7/2
  Product21/1 -> Gain4/1  "prod"
  Demux30/1 -> Mux37/1  "Product_a_proposed"
  [Yabc] -> Scope13/3, Product22/2
  [Y_DQN_vec] -> Mult_DQN4/2, Mult_DQN3/2
  MATLAB Function1/5(z5) -> Add7/5
  Demux29/3 -> Mux39/2  "Product_c_ref"
  [Xabc] -> Subtract1/2  "prod"
  Mux37/1 -> XY7/1
  [th0] -> sDQN2abc10/2
  sInt_DQN4/1 -> Scope14/2, Mult_DQN4/1  "Vp_M"
  Product18/1 -> Discrete-Time Integrator4/1  "dVp_M"
  sMult_DQN2/1(Out1) -> sInt_DQN1/1
  Delay2/1 -> Add10/2
  Subtract/1 -> Product22/1
  [Xabc] -> MATLAB Function2/1(x)  "prod"
  [Xabc] -> Product20/1
  Discrete-Time Integrator5/1 -> Scope13/1, Subtract/1  "Vp_M"
  MATLAB Function1/4(z4) -> Add7/4
  Product22/1 -> Discrete-Time Integrator5/1  "dVp_M"
  MATLAB Function1/1(z1) -> Add7/1
  MATLAB Function2/1(z) -> Gain9/1
  Gain5/1 -> Int/1(x)
  Discrete-Time Integrator4/1 -> Product19/1  "Vp_M"
  Add10/1 -> Add11/1, Gain5/1
  sAdd_DQN2/1(Out1) -> sMult_DQN2/1(In1)
  Delay4/1 -> Add10/4
  Gain3/1 -> sAdd_DQN3/1(In1)
  Int/1(z) -> Scope11/3, Scope10/2, Delay3/1, Scope10/1
  Add7/1 -> Scope11/2
  MATLAB Function1/3(z3) -> Add7/3
  [Yabc] -> Product21/1, Product20/2
  Product20/1 -> Gain1/1  "prod"
  sInt_DQN1/1 -> Delay/1, Reshape/1, sDQN2abc8/1
  Demux21/1 -> Mux28/1  "Product_a_proposed"
  sInt_DQN2/1 -> Delay1/1, sDQN2abc9/1
  From52/1 -> sMult_DQN3/2(In2)
  From50/1 -> sAdd_DQN3/2(In2)
  From53/1 -> sDQN2abc9/2
  Gain2/1 -> sAdd_DQN2/1(In1)
  Delay1/1 -> Subsystem1/1("{X_DQN}")
  sMult_DQN3/1(Out1) -> sInt_DQN2/1
  [Xabc] -> MATLAB Function1/1(x), Add5/2
  From44/1 -> sAdd_DQN2/2(In2)
  [Yabc] -> Product17/2, MATLAB Function1/2(y)
  Demux21/2 -> Mux29/1  "Product_b_proposed"
  Subsystem3/1("{Y_DQN}") -> Gain34/1
  Add5/1 -> Product17/1
  Delay/1 -> Subsystem2/1("{X_DQN}")
  From48/1 -> sDQN2abc8/2
  Demux18/1 -> Mux28/2  "Product_a_ref"
  Product19/1 -> Discrete-Time Integrator6/1
  Demux18/2 -> Mux29/2  "Product_b_ref"
  Demux21/3 -> Mux31/1  "Product_c_proposed"
  Discrete-Time Integrator6/1 -> Demux30/1, Gain7/1  "Vp_M"
  Mux31/1 -> XY4/3
  Mux28/1 -> XY4/1
  sDQN2abc8/1 -> Demux21/1
  Demux28/1 -> Mux28/3  "Product_a_ref"
  Mux29/1 -> XY4/2
  Delay3/1 -> Product21/2, Add11/2
  Subsystem2/1("{Y_DQN}") -> Gain2/1
  Demux18/3 -> Mux31/2  "Product_c_ref"
  Delay5/1 -> Subsystem3/1("{X_DQN}")
  Reshape/1 -> Display/1
  Gain7/1 -> Subtract1/1  "dVp_M"
  MATLAB Function1/2(z2) -> Add7/2
  Demux30/2 -> Mux38/1  "Product_b_proposed"
  Gain1/1 -> Delay2/1, Add10/1
  Gain4/1 -> Delay4/1, Add10/3
  Discrete-Time Integrator3/1 -> Add5/1, Demux28/1, Scope11/1
  Demux29/1 -> Mux37/2  "Product_a_ref"
  From24/1 -> Mult_DQN2/1(X_DQN)
  Mult_DQN2/1(Z_DQN) -> Reshape5/1, DQN2abc5/1
  Demux9/2 -> Mux14/1  "Product_b_proposed"
  From/1 -> sAdd_DQN/1
  Add/1 -> Demux8/1
  Demux17/2 -> Mux24/1  "Product_b_proposed"
  Mux14/1 -> XY2/2
  Demux17/1 -> Mux23/1  "Product_a_proposed"
  From36/1 -> Product10/2
  From35/1 -> Product10/1
  Product10/1 -> Demux16/1  "prod"
  From30/1 -> Product10/3
  Demux8/3 -> Mux18/2  "Product_c_ref"
  Product8/1 -> Add/1
  From22/1 -> Add/2, Product8/2
  Reshape5/1 -> Display1/1
  Mux25/1 -> XY6/3
  DQN2abc5/1 -> Demux17/1
  From34/1 -> Mult_DQN2/2(Y_DQN)
  Demux8/1 -> Mux13/2  "Product_a_ref"
  Demux16/1 -> Mux23/2  "Product_a_ref"
  Demux16/2 -> Mux24/2  "Product_b_ref"
  Demux16/3 -> Mux25/2  "Product_c_ref"
  Mux23/1 -> XY6/1
  Demux9/1 -> Mux13/1  "Product_a_proposed"
  From18/1 -> sAdd_DQN/2
  From33/1 -> DQN2abc5/2
  From17/1 -> Product8/1
  From21/1 -> sDQN2abc3/2
  Demux8/2 -> Mux14/2  "Product_b_ref"
  Mux24/1 -> XY6/2
  Mux18/1 -> XY2/3
  sDQN2abc3/1 -> Demux9/1
  Mux13/1 -> XY2/1
  sAdd_DQN/1 -> sDQN2abc3/1
  Demux17/3 -> Mux25/1  "Product_c_proposed"
  Demux9/3 -> Mux18/1  "Product_c_proposed"

== system DQN_ABC_Test/Subsystem/Mult_DQN2 ==
  X_DQN : Inport
  Y_DQN : Inport  Port=2
  DQn (Full)10 : MATLAB Function  TreatAsAtomicUnit=on  mask{N=HrmOrd, HrmDbl=HrmDbl, chkHrmLst=chkHrmLst, HrmLstX=HrmLstX, HrmLstY=HrmLstY}
      mask prompts: N "Harmonic order:"; HrmDbl "Double Harmonic"; chkHrmLst "Only specific harmonics:"; HrmLstX "Harmonic list X:"; HrmLstY "Harmonic list Y:"
  Demux : Demux  Outputs=6
  Demux1 : Demux  Outputs=6
  Mux51 : Mux  Inputs=[(HrmDbl+1)*HrmOrd+1,(HrmDbl+1)*HrmOrd+1,(HrmDbl+1)*HrmOrd+1,(HrmDbl+1)*HrmOrd+1,(HrmDbl+1)*HrmOrd+1,(HrmDbl+1)*HrmOrd+1]
  Z_DQN : Outport
  wires:
  DQn (Full)10/6(Zqz) -> Mux51/6
  DQn (Full)10/5(Zqn) -> Mux51/5
  DQn (Full)10/1(Zdp) -> Mux51/1
  DQn (Full)10/4(Zqp) -> Mux51/4
  DQn (Full)10/2(Zdn) -> Mux51/2
  DQn (Full)10/3(Zdz) -> Mux51/3
  Demux1/6 -> DQn (Full)10/12(Yqz)
  Demux1/5 -> DQn (Full)10/11(Yqn)
  Demux1/4 -> DQn (Full)10/10(Yqp)
  Demux1/3 -> DQn (Full)10/9(Ydz)
  Demux1/2 -> DQn (Full)10/8(Ydn)
  Demux1/1 -> DQn (Full)10/7(Ydp)
  Demux/6 -> DQn (Full)10/6(Xqz)
  Demux/5 -> DQn (Full)10/5(Xqn)
  Demux/4 -> DQn (Full)10/4(Xqp)
  Demux/3 -> DQn (Full)10/3(Xdz)
  Demux/2 -> DQn (Full)10/2(Xdn)
  Demux/1 -> DQn (Full)10/1(Xdp)
  Mux51/1 -> Z_DQN/1
  Y_DQN/1 -> Demux1/1
  X_DQN/1 -> Demux/1

== system DQN_ABC_Test/Subsystem/Subsystem1 ==
  "{X_DQN}" : Inport
  Demux28 : Demux  Outputs=[Hi+1,Hi+1,Hi+1,Hi+1,Hi+1,Hi+1]
  Mux : Mux  Inputs=[Ho+1,Ho+1,Ho+1,Ho+1,Ho+1,Ho+1]
  Selector{,1..5} (6 alike) : Selector  InputPortWidth=Hi+1  IndexOptions=Index vector (dialog)  Indices=[1:Ho+1]  OutputSizes=1
  "{Y_DQN}" : Outport
  wires:
  Selector5/1 -> Mux/6
  Selector2/1 -> Mux/3
  Demux28/2 -> Selector1/1
  Demux28/1 -> Selector/1
  Demux28/3 -> Selector2/1
  Selector/1 -> Mux/1
  Demux28/4 -> Selector3/1
  Selector1/1 -> Mux/2
  Selector3/1 -> Mux/4
  "{X_DQN}"/1 -> Demux28/1
  Selector4/1 -> Mux/5
  Demux28/5 -> Selector4/1
  Demux28/6 -> Selector5/1
  Mux/1 -> "{Y_DQN}"/1

== system DQN_ABC_Test/Subsystem/Subsystem2 ==
  "{X_DQN}" : Inport
  Demux28 : Demux  Outputs=[Hi+1,Hi+1,Hi+1,Hi+1,Hi+1,Hi+1]
  Mux : Mux  Inputs=[Ho+1,Ho+1,Ho+1,Ho+1,Ho+1,Ho+1]
  Selector{,1..5} (6 alike) : Selector  InputPortWidth=Hi+1  IndexOptions=Index vector (dialog)  Indices=[1:Ho+1]  OutputSizes=1
  "{Y_DQN}" : Outport
  wires:
  Selector5/1 -> Mux/6
  Selector2/1 -> Mux/3
  Demux28/2 -> Selector1/1
  Demux28/1 -> Selector/1
  Demux28/3 -> Selector2/1
  Selector/1 -> Mux/1
  Demux28/4 -> Selector3/1
  Selector1/1 -> Mux/2
  Selector3/1 -> Mux/4
  "{X_DQN}"/1 -> Demux28/1
  Selector4/1 -> Mux/5
  Demux28/5 -> Selector4/1
  Demux28/6 -> Selector5/1
  Mux/1 -> "{Y_DQN}"/1

== system DQN_ABC_Test/Subsystem/Subsystem3 ==
  "{X_DQN}" : Inport
  Demux28 : Demux  Outputs=[Hi+1,Hi+1,Hi+1,Hi+1,Hi+1,Hi+1]
  Mux : Mux  Inputs=[Ho+1,Ho+1,Ho+1,Ho+1,Ho+1,Ho+1]
  Selector{,1..5} (6 alike) : Selector  InputPortWidth=Hi+1  IndexOptions=Index vector (dialog)  Indices=[1:Ho+1]  OutputSizes=1
  "{Y_DQN}" : Outport
  wires:
  Selector5/1 -> Mux/6
  Selector2/1 -> Mux/3
  Demux28/2 -> Selector1/1
  Demux28/1 -> Selector/1
  Demux28/3 -> Selector2/1
  Selector/1 -> Mux/1
  Demux28/4 -> Selector3/1
  Selector1/1 -> Mux/2
  Selector3/1 -> Mux/4
  "{X_DQN}"/1 -> Demux28/1
  Selector4/1 -> Mux/5
  Demux28/5 -> Selector4/1
  Demux28/6 -> Selector5/1
  Mux/1 -> "{Y_DQN}"/1

== system DQN_ABC_Test/Subsystem/sAdd_DQN2 ==
  In1 : Inport
  In2 : Inport  Port=2
  Demux : Demux  Outputs=[HRM+1,HRM+1,HRM+1,HRM+1,HRM+1,HRM+1]
  Demux7 : Demux  Outputs=[HRM+1,HRM+1,HRM+1,HRM+1,HRM+1,HRM+1]
  Mux7 : Mux  Inputs=[HRM+1,HRM+1,HRM+1,HRM+1,HRM+1,HRM+1]
  S-Function : S-Function  FunctionName=sAddDQN  Parameters=HRM  SFunctionDeploymentMode=off  EnableBusSupport=off  mask{HRM=HRM}
      mask prompts: HRM "Harmonic order:"
  Out1 : Outport
  wires:
  In1/1 -> Demux/1
  Demux/1 -> S-Function/1
  Demux7/2 -> S-Function/8
  Demux7/6 -> S-Function/12
  Demux/5 -> S-Function/5
  Demux7/4 -> S-Function/10
  Demux7/1 -> S-Function/7
  Demux/4 -> S-Function/4
  Demux7/3 -> S-Function/9
  Mux7/1 -> Out1/1
  Demux/6 -> S-Function/6
  In2/1 -> Demux7/1
  Demux/2 -> S-Function/2
  S-Function/2 -> Mux7/2
  Demux/3 -> S-Function/3
  S-Function/1 -> Mux7/1
  S-Function/5 -> Mux7/5
  Demux7/5 -> S-Function/11
  S-Function/3 -> Mux7/3
  S-Function/4 -> Mux7/4
  S-Function/6 -> Mux7/6

== system DQN_ABC_Test/Subsystem/sAdd_DQN3 ==
  In1 : Inport
  In2 : Inport  Port=2
  Demux : Demux  Outputs=[HRM+1,HRM+1,HRM+1,HRM+1,HRM+1,HRM+1]
  Demux7 : Demux  Outputs=[HRM+1,HRM+1,HRM+1,HRM+1,HRM+1,HRM+1]
  Mux7 : Mux  Inputs=[HRM+1,HRM+1,HRM+1,HRM+1,HRM+1,HRM+1]
  S-Function : S-Function  FunctionName=sAddDQN  Parameters=HRM  SFunctionDeploymentMode=off  EnableBusSupport=off  mask{HRM=HRM}
      mask prompts: HRM "Harmonic order:"
  Out1 : Outport
  wires:
  In1/1 -> Demux/1
  Demux/1 -> S-Function/1
  Demux7/2 -> S-Function/8
  Demux7/6 -> S-Function/12
  Demux/5 -> S-Function/5
  Demux7/4 -> S-Function/10
  Demux7/1 -> S-Function/7
  Demux/4 -> S-Function/4
  Demux7/3 -> S-Function/9
  Mux7/1 -> Out1/1
  Demux/6 -> S-Function/6
  In2/1 -> Demux7/1
  Demux/2 -> S-Function/2
  S-Function/2 -> Mux7/2
  Demux/3 -> S-Function/3
  S-Function/1 -> Mux7/1
  S-Function/5 -> Mux7/5
  Demux7/5 -> S-Function/11
  S-Function/3 -> Mux7/3
  S-Function/4 -> Mux7/4
  S-Function/6 -> Mux7/6

== system DQN_ABC_Test/Subsystem/sMult_DQN2 ==
  In1 : Inport
  In2 : Inport  Port=2
  Demux : Demux  Outputs=[HRM+1,HRM+1,HRM+1,HRM+1,HRM+1,HRM+1]
  Demux7 : Demux  Outputs=[HRM+1,HRM+1,HRM+1,HRM+1,HRM+1,HRM+1]
  Mux7 : Mux  Inputs=[(HrmDbl+1)*HRM+1,(HrmDbl+1)*HRM+1,(HrmDbl+1)*HRM+1,(HrmDbl+1)*HRM+1,(HrmDbl+1)*HRM+1,(HrmDbl+1)*HRM+1]
  S-Function : S-Function  FunctionName=sMultDQN  Parameters=HRM chkHrm  SFunctionDeploymentMode=off  EnableBusSupport=off  mask{HRM=HRM, chkHrm=HrmOpt}
      mask prompts: HRM "Harmonic order:"; chkHrm "Double harmonic:"
  Out1 : Outport
  wires:
  In1/1 -> Demux/1
  Demux/1 -> S-Function/1
  Demux7/2 -> S-Function/8
  Demux7/6 -> S-Function/12
  Demux/5 -> S-Function/5
  Demux7/4 -> S-Function/10
  Demux7/1 -> S-Function/7
  Demux/4 -> S-Function/4
  Demux7/3 -> S-Function/9
  Mux7/1 -> Out1/1
  Demux/6 -> S-Function/6
  In2/1 -> Demux7/1
  Demux/2 -> S-Function/2
  S-Function/2 -> Mux7/2
  Demux/3 -> S-Function/3
  S-Function/1 -> Mux7/1
  S-Function/5 -> Mux7/5
  Demux7/5 -> S-Function/11
  S-Function/3 -> Mux7/3
  S-Function/4 -> Mux7/4
  S-Function/6 -> Mux7/6

== system DQN_ABC_Test/Subsystem/sMult_DQN3 ==
  In1 : Inport
  In2 : Inport  Port=2
  Demux : Demux  Outputs=[HRM+1,HRM+1,HRM+1,HRM+1,HRM+1,HRM+1]
  Demux7 : Demux  Outputs=[HRM+1,HRM+1,HRM+1,HRM+1,HRM+1,HRM+1]
  Mux7 : Mux  Inputs=[(HrmDbl+1)*HRM+1,(HrmDbl+1)*HRM+1,(HrmDbl+1)*HRM+1,(HrmDbl+1)*HRM+1,(HrmDbl+1)*HRM+1,(HrmDbl+1)*HRM+1]
  S-Function : S-Function  FunctionName=sMultDQN  Parameters=HRM chkHrm  SFunctionDeploymentMode=off  EnableBusSupport=off  mask{HRM=HRM, chkHrm=HrmOpt}
      mask prompts: HRM "Harmonic order:"; chkHrm "Double harmonic:"
  Out1 : Outport
  wires:
  In1/1 -> Demux/1
  Demux/1 -> S-Function/1
  Demux7/2 -> S-Function/8
  Demux7/6 -> S-Function/12
  Demux/5 -> S-Function/5
  Demux7/4 -> S-Function/10
  Demux7/1 -> S-Function/7
  Demux/4 -> S-Function/4
  Demux7/3 -> S-Function/9
  Mux7/1 -> Out1/1
  Demux/6 -> S-Function/6
  In2/1 -> Demux7/1
  Demux/2 -> S-Function/2
  S-Function/2 -> Mux7/2
  Demux/3 -> S-Function/3
  S-Function/1 -> Mux7/1
  S-Function/5 -> Mux7/5
  Demux7/5 -> S-Function/11
  S-Function/3 -> Mux7/3
  S-Function/4 -> Mux7/4
  S-Function/6 -> Mux7/6

== matlab function DQN_ABC_Test/Subsystem/MATLAB Function ==
  data: Xdp input; Xdn input; Xdz input; Xqp input; Xqn input; Xqz input; Zdp output; hIn parameter; hOut parameter; Zdn output; Zdz output; Zqp output; Zqn output; Zqz output
function [Zdp,Zdn,Zdz,Zqp,Zqn,Zqz]  = TrimDQN(Xdp, Xdn, Xdz, Xqp, Xqn, Xqz, hIn, hOut)


Zdp = Xdp(1:hOut);
Zdn = Xdn(1:hOut);
Zdz = Xdz(1:hOut);
Zqp = Xqp(1:hOut);
Zqn = Xqn(1:hOut);
Zqz = Xqz(1:hOut);
% 
% function y = fcn(u, hIn, hOut)
% Off = (hIn+1);
% y = u([0*Off+1:hOut+1,Off+1:Off+hOut+1,2*Off+1:2*Off+hOut+1,3*Off+1:3*Off+hOut+1,4*Off+1:4*Off+hOut+1,5*Off+1:5*Off+hOut+1]);

== matlab function DQN_ABC_Test/MATLAB Function4 ==
  data: Xpnz input; Xabc output; th input; HRM parameter; X_DQN output; chkHrmLst parameter; HrmLst parameter
function [Xabc, X_DQN] = fcn(Xpnz, th, HRM, chkHrmLst, HrmLst)
abc3p = zeros(3,1);

    X_DQN = zeros((HRM+1)*6,1);
    
    if(chkHrmLst)
        range = numel(HrmLst);
    else
       range = HRM+1; 
       
    end
    
    h = 0;
    for i = 1:range
        
        if(chkHrmLst)
            h = HrmLst(i)+1;
        else
            h = i; 
        end
        
        Magp = Xpnz(1,h);
        Angp = Xpnz(2,h);
        Magn = Xpnz(3,h);
        Angn = Xpnz(4,h);
        Magz = Xpnz(5,h);
        Angz = Xpnz(6,h);

        Xdp = Magp*cos(Angp);
        Xqp = Magp*sin(Angp);
        Xdn =-Magn*cos(Angn);
        Xqn = Magn*sin(Angn);
        Xdz = Magz*cos(Angz);
        Xqz = Magz*sin(Angz);

        Tda_p = [sin((h-1)*th)            cos((h-1)*th);
                 sin((h-1)*th-2*pi/3)     cos((h-1)*th-2*pi/3);
                 sin((h-1)*th+2*pi/3)     cos((h-1)*th+2*pi/3)];

        Tda_n = [sin(-(h-1)*th)           cos(-(h-1)*th);
                 sin(-(h-1)*th-2*pi/3)    cos(-(h-1)*th-2*pi/3);
                 sin(-(h-1)*th+2*pi/3)    cos(-(h-1)*th+2*pi/3)];

        Tda_z = [sin((h-1)*th)            cos((h-1)*th);
                 sin((h-1)*th)            cos((h-1)*th);
                 sin((h-1)*th)            cos((h-1)*th)];


        Tdqn_a = [Tda_p(:,1)  Tda_n(:,1)  Tda_z(:,1)  Tda_p(:,2)  Tda_n(:,2)  Tda_z(:,2)];

        if(h==1)
            abc3p = abc3p + Tdqn_a*[Xdp;-Xdn;Xdz;Xqp;Xqn;Xqz];
            
            X_DQN(h+0*(HRM+1)) = 2*Xdp;
            X_DQN(h+1*(HRM+1)) = -2*Xdn;
            X_DQN(h+2*(HRM+1)) = 0;
            X_DQN(h+3*(HRM+1)) = 2*Xqp;
            X_DQN(h+4*(HRM+1)) = 2*Xqn;
            X_DQN(h+5*(HRM+1)) = Xqz;
            
        else
            abc3p = abc3p + Tdqn_a*[Xdp;Xdn;Xdz;Xqp;Xqn;Xqz];
            
            X_DQN(h+0*(HRM+1)) = Xdp;
            X_DQN(h+1*(HRM+1)) = Xdn;
            X_DQN(h+2*(HRM+1)) = Xdz;
            X_DQN(h+3*(HRM+1)) = Xqp;
            X_DQN(h+4*(HRM+1)) = Xqn;
            X_DQN(h+5*(HRM+1)) = Xqz;
        end
        


    end


    Xabc = abc3p;
    
end

== matlab function DQN_ABC_Test/Subsystem/MATLAB Function1 ==
  settings: updateMethod=DISCRETE
  data: x input; z1 output; y input; z2 output; z3 output; z4 output; z5 output
function [z1,z2,z3,z4,z5] = fcn(x,y)

    dt = 5.0000e-06;
    z = zeros(3,1);
    z1 = zeros(3,1);
    z2 = zeros(3,1);
    z3 = zeros(3,1);
    z4 = zeros(3,1);
    z5 = zeros(3,1);

    persistent z_o;    
    persistent z_o2;
    persistent y_o;
    persistent x_o;   
    persistent dt2;
    
    if(isempty(dt2))
        dt2     = dt/2; 
        z_o     = zeros(3,1);
        z_o2    = zeros(3,1);
        x_o     = zeros(3,1);
        y_o     = zeros(3,1);    
    end

    z1 = dt2*x.*y;
    z2 = dt2*x_o.*y_o;
    z3 = -dt2*z_o.*y;
    z4 = -dt2*z_o2.*y_o;
    z5 = z_o;
    
    z = z1+z2+z3+z4+z5;

    x_o = x;
    y_o = y;
    z_o2 = z_o;
    z_o = z;
    
    
    
end

== matlab function DQN_ABC_Test/Subsystem/Int ==
  settings: updateMethod=DISCRETE
  data: x input; z output; dt parameter
function z = fcn(x, dt)

    persistent z_old;    
    persistent x_old;   
    persistent dt2;
    
    if(isempty(dt2))
        dt2 = dt/2; 
        z_old  = zeros(3,1);
        x_old  = zeros(3,1);
    end
    
    R = -1;
    iL = 1;
    Krl1 = (dt2*iL/(1+dt2*R*iL));
    Krl2 = (1-dt2*R*iL)/(1+dt2*R*iL);
    
    z = zeros(3,1);

    %z = (dt2)*(x+x_old)+z_old;
    z = Krl1*(x+x_old)+Krl2*z_old;
    z_old = z;
    x_old = x;
    
end

== matlab function DQN_ABC_Test/Subsystem/MATLAB Function2 ==
  data: x input; z output; y input
function z  = fcn(x,y)

    dt = 5.0000e-06;
    z = zeros(3,1);
    e = zeros(3,1);


    persistent dt2;
    persistent eo;
    persistent xo;
    persistent yo;
    persistent zo;
    
    
    if(isempty(dt2))
        dt2     = dt/2; 
        xo = zeros(3,1);
        yo = zeros(3,1);
        eo = zeros(3,1);
    end
    

    z = dt*(xo.*yo.^2)+eo.*yo;
    xo = x;
    yo = y;
    eo = eo + dt*(xo.*yo);
    
    %z = e.*y;
    
end

== matlab function DQN_ABC_Test/MATLAB Function8 ==
  data: Xpnz_ci input; Xabc output; tho input; HRM parameter; Xpnz_c output
function [Xabc,Xpnz_c] = fcn(Xpnz_ci, tho, HRM)

Xabc = zeros(3,1);


a = -0.5+0.866i;
a2 = -0.5-0.866i;
Sas = [1,a,a2;1,a2,a;1,1,1]/3;
Ssa = inv(Sas);

for i = 1 : HRM+1


    if(i>1)
        h = i-1;

        th = h*tho;
    
        mag_p = abs(Xpnz_ci(1,i));
        ang_p = angle(Xpnz_ci(1,i));
        mag_n = abs(Xpnz_ci(2,i));
        ang_n = angle(Xpnz_ci(2,i));
        mag_z = abs(Xpnz_ci(3,i));
        ang_z = angle(Xpnz_ci(3,i));
        
        abc3p = mag_p*[sin(th+ang_p) ; sin(th+ang_p-2*pi/3) ; sin(th+ang_p+2*pi/3) ];
        abc3n = mag_n*[sin(th+ang_n) ; sin(th+ang_n+2*pi/3) ; sin(th+ang_n-2*pi/3) ];
        abc3z = mag_z*[sin(th+ang_z) ; sin(th+ang_z)        ; sin(th+ang_z)  ];
    
        Xabc = Xabc + abc3p+abc3n+abc3z;
    else
        Xabc = Xabc + real(Ssa*(Xpnz_ci(:,1)));
    
    end

Xpnz_c = Xpnz_ci;
    
end
